simulink model "Demo1"  (Simulink 7.7)
settings: Solver=ode45  StartTime=0.0  StopTime=10  RelTol=1e-3
PreLoadFcn:
  | EbNo = 16; Errors = 188; Bits = 1e8; M = 256; N = 64; Ts = 1/22050; InnerInterleaverBitTable;constellation;
undefined symbols (not defined in the file or in its folder): gray, Rec, rsgenpoly, SDTV, sz
libraries: vipmisc x22, dspsigops x9, commutil2 x8, viptransforms x6, viputilities x6, vipconversions x4, dspobslib x4, commblkintrlv2 x4, commblkcod2 x2, vipsnks x2, commcnvintrlv2 x2, commsink2 x2
(part 2 of 2)

== system Demo1/Audio Source/Encoder/Block Processing/Block iterator/sub-block process/Transform coder2 ==
  In1 : Inport
  2D DCT : viptransforms/2-D DCT  CompMethod=Table lookup  Dimension=0  TableOpt=Speed  BitRevOrder=off  SkipNorm=off  firstCoeffDataTypeStr=Inherit: Same word length as input  firstCoeffLastDataTypeStr=Inherit: Same word length as input  outputMin=[]  outputMax=[]  roundingMode=Floor  overflowMode=off
  AC zigzag : Selector  IndexOptions=Index vector (dialog)  Indices="([0  8     1     2     9    16    24    17    10     3     4    11    18    25  32    40    33    26    19    12     5     6    13    20    27    34    41  48    56    49    42    35    28    21    14     7    15    22    29    36  43    50    57    58    51    44    37    30    23    31    38    45    52  59    60    53    46    39    47    54    61    62    55    63]+1)"  OutputSizes=1
  Bit Pack : Stateflow chart  TreatAsAtomicUnit=on
  Gain : Gain  Gain=255/8
  Gain1 : Gain  Gain=255/8
  Matrix Concatenation : Concatenate  Mode=Multidimensional array
  Reshape : Reshape  OutputDimensionality=Column vector (2-D)  OutputDimensions=[8,8]
  Reshape1 : Reshape  OutputDimensionality=Column vector (2-D)  OutputDimensions=[8,8]
  select 0 : Selector  IndexMode=Zero-based  IndexOptions=Index vector (dialog)  Indices=(0)  OutputSizes=8,8
  select 1 : Selector  IndexMode=Zero-based  IndexOptions=Starting index (dialog)  Indices=(1)  OutputSizes=63
  Out1 : Outport
  wires:
  Gain1/1 -> Matrix Concatenation/2
  select 1/1 -> Gain1/1
  Gain/1 -> Matrix Concatenation/1
  Matrix Concatenation/1 -> AC zigzag/1
  select 0/1 -> Gain/1
  Reshape/1 -> select 1/1, select 0/1
  Reshape1/1 -> Out1/1
  2D DCT/1 -> Reshape/1
  In1/1 -> 2D DCT/1
  AC zigzag/1 -> Bit Pack/1(in)
  Bit Pack/1(out) -> Reshape1/1

== system Demo1/Audio Sink/Decoder/Block Processing/Block iterator/sub-block process/Motion compensation decoder/SelectMatch3 ==
  Image : Inport
  Indx : Inport  Port=2
  Selector3 : Selector  NumberOfDimensions=2  IndexMode=Zero-based  InputPortWidth=3  IndexOptions=Starting index (port),Starting index (port)  Indices=1,1  OutputSizes=16, 16
  Selector4 : Selector  InputPortWidth=2  IndexOptions=Index vector (dialog)  Indices=1  OutputSizes=1
  Selector5 : Selector  InputPortWidth=2  IndexOptions=Index vector (dialog)  Indices=2  OutputSizes=1
  Out : Outport
  wires:
  Selector3/1 -> Out/1
  Indx/1 -> Selector5/1, Selector4/1
  Image/1 -> Selector3/1
  Selector5/1 -> Selector3/3
  Selector4/1 -> Selector3/2

== system Demo1/Audio Sink/Decoder/Block Processing/Block iterator/sub-block process/Motion compensation decoder/SelectMatch4 ==
  Image : Inport
  Indx : Inport  Port=2
  Selector3 : Selector  NumberOfDimensions=2  IndexMode=Zero-based  InputPortWidth=3  IndexOptions=Starting index (port),Starting index (port)  Indices=1,1  OutputSizes=8, 8
  Selector4 : Selector  InputPortWidth=2  IndexOptions=Index vector (dialog)  Indices=1  OutputSizes=1
  Selector5 : Selector  InputPortWidth=2  IndexOptions=Index vector (dialog)  Indices=2  OutputSizes=1
  Out : Outport
  wires:
  Selector4/1 -> Selector3/2
  Selector5/1 -> Selector3/3
  Image/1 -> Selector3/1
  Indx/1 -> Selector4/1, Selector5/1
  Selector3/1 -> Out/1

== system Demo1/Audio Sink/Decoder/Block Processing/Block iterator/sub-block process/Motion compensation decoder/SelectMatch5 ==
  Image : Inport
  Indx : Inport  Port=2
  Selector3 : Selector  NumberOfDimensions=2  IndexMode=Zero-based  InputPortWidth=3  IndexOptions=Starting index (port),Starting index (port)  Indices=1,1  OutputSizes=8, 8
  Selector4 : Selector  InputPortWidth=2  IndexOptions=Index vector (dialog)  Indices=1  OutputSizes=1
  Selector5 : Selector  InputPortWidth=2  IndexOptions=Index vector (dialog)  Indices=2  OutputSizes=1
  Out : Outport
  wires:
  Selector3/1 -> Out/1
  Indx/1 -> Selector5/1, Selector4/1
  Image/1 -> Selector3/1
  Selector5/1 -> Selector3/3
  Selector4/1 -> Selector3/2

== system Demo1/Audio Source/Encoder/Block Processing/Block iterator/sub-block process/Motion compensation encoder/SelectMatch ==
  Image : Inport
  Indx : Inport  Port=2
  Selector3 : Selector  NumberOfDimensions=2  IndexMode=Zero-based  InputPortWidth=3  IndexOptions=Starting index (port),Starting index (port)  Indices=(1),(1)  OutputSizes=16,16
  Selector4 : Selector  InputPortWidth=2  IndexOptions=Index vector (dialog)  Indices=(1)  OutputSizes=1
  Selector5 : Selector  InputPortWidth=2  IndexOptions=Index vector (dialog)  Indices=(2)  OutputSizes=1
  Out : Outport
  wires:
  Selector4/1 -> Selector3/2
  Selector5/1 -> Selector3/3
  Image/1 -> Selector3/1
  Indx/1 -> Selector4/1, Selector5/1
  Selector3/1 -> Out/1

== system Demo1/Audio Source/Encoder/Block Processing/Block iterator/sub-block process/Motion compensation encoder/SelectMatch1 ==
  Image : Inport
  Indx : Inport  Port=2
  Selector3 : Selector  NumberOfDimensions=2  IndexMode=Zero-based  InputPortWidth=3  IndexOptions=Starting index (port),Starting index (port)  Indices=(1),(1)  OutputSizes=8,8
  Selector4 : Selector  InputPortWidth=2  IndexOptions=Index vector (dialog)  Indices=(1)  OutputSizes=1
  Selector5 : Selector  InputPortWidth=2  IndexOptions=Index vector (dialog)  Indices=(2)  OutputSizes=1
  Out : Outport
  wires:
  Selector3/1 -> Out/1
  Indx/1 -> Selector5/1, Selector4/1
  Image/1 -> Selector3/1
  Selector5/1 -> Selector3/3
  Selector4/1 -> Selector3/2

== system Demo1/Audio Source/Encoder/Block Processing/Block iterator/sub-block process/Motion compensation encoder/SelectMatch2 ==
  Image : Inport
  Indx : Inport  Port=2
  Selector3 : Selector  NumberOfDimensions=2  IndexMode=Zero-based  InputPortWidth=3  IndexOptions=Starting index (port),Starting index (port)  Indices=(1),(1)  OutputSizes=8,8
  Selector4 : Selector  InputPortWidth=2  IndexOptions=Index vector (dialog)  Indices=(1)  OutputSizes=1
  Selector5 : Selector  InputPortWidth=2  IndexOptions=Index vector (dialog)  Indices=(2)  OutputSizes=1
  Out : Outport
  wires:
  Selector4/1 -> Selector3/2
  Selector5/1 -> Selector3/3
  Image/1 -> Selector3/1
  Indx/1 -> Selector4/1, Selector5/1
  Selector3/1 -> Out/1

== matlab function Audio Source/Encoder/Block Processing/Block iterator/sub-block process/Transform coder/Bit Pack ==
  data: in input double; out output uint32 size=20
function out=bitpack(in) 

% Pack output bits into given length using run length coding. The first 
% coefficient (DC) is coded using 32 bits. The AC coefficients are run 
% length coded using 4 bits for run and 8 bits for value. The output is uint32.

persistent prev_out;
if isempty(prev_out)
    prev_out = uint32(zeros(20,1));
end
    out=uint32(prev_out);
    % Bit Pack Routine  
    bitpos=int32(0); 
    Temp= uint32(0); 
    run =  uint32(0); 
    outpos = 2; 
    pval=single(0); 
    cval=single(0);
  
    numcoefs = 64;
    
    out1 =  int32(fix(in(1)));
    
    if out1>=-1   
       out(1) = uint32(out1);
    else
       out(1) = uint32(intmax('uint32') - uint32(abs(out1)) +uint32(2));
    end

    % ac coefficients
    % 4 bit - run length followed by 8 bit coef value  
    pval(:) = fix(in(2)+0.5);
    if (pval > 127),  pval(:) = 127; end % saturate  
    if (pval < -128), pval(:) = -128; end

    run(:) = 0;
    for i=(3): numcoefs   
        cval(:) = floor(in(i)+0.5); 
        if (pval == cval && run < 14)  
            run(:)=run(:)+1;
        else  
            [flag, bitpos, out, Temp, outpos] = putbits(bitpos, out, Temp, outpos, run, 4);
            if (~flag) 
                prev_out=out;
                return; 
            end

            if (pval > 127),  pval(:) = 127;  end % saturate  
            if (pval < -128), pval(:) = -128; end
            pval(:) = pval+128; % make positive  

            [flag, bitpos, out, Temp, outpos] = putbits(bitpos, out, Temp, outpos, uint32(pval), 8);
            if (~flag) 
                prev_out=out;
                return; 
            end

            run(:) = 0;
        end
        pval(:) = cval;
    end

    % last coefficient  
    [flag, bitpos, out, Temp, outpos] = putbits(bitpos, out, Temp, outpos, run, 4);
    if (~flag) 
        prev_out=out;
        return; 
    end

    if (pval > 127),  pval(:) = 127;  end % saturate 
    if (pval < -128), pval(:) = -128; end
    pval(:) = pval+128; % make positive 

    [flag, bitpos, out, Temp, outpos] = putbits(bitpos, out, Temp, outpos, pval, 8);
    if (~flag) 
        prev_out=out;
        return; 
    end

    [bitpos, out, Temp, outpos] = flushbits(bitpos, out, Temp, outpos);%#ok
    prev_out=out;
end

%%========================================================================
function [flag, bitposO, outO, TempO, outposO] = putbits(bitpos, out, Temp, outpos, val, bits)
     
    valIn = uint32(val);
    bitsIn=int32(bits);
    bitposO = int32(bitpos);
    outO = uint32(out);
    TempO = uint32(Temp);
    outposO = outpos;
    
    if (bitposO + bitsIn > 32)  
        bitsleft = int32(32 - bitposO);
        bval=uint32(0);
        bval(:) = bitshift(valIn, -(bitsIn-bitsleft)); 
        TempO(:) = bitor(TempO,bval); 
        outO(outposO) = TempO;
        outposO = outposO+1;
        if (outposO > length(out))  
            flag = 0;
            return;
        end
        TempO = uint32(0);
        bitposO(:) = int32(0);
        bitsIn(:) = bitsIn-bitsleft; 
        valIn(:)=bitshift(valIn, 32-bitsIn);  
        valIn(:)=bitshift(valIn, -(32-bitsIn)); 
    end
    valIn(:)=bitshift(valIn, (32-(bitsIn+(bitposO))));  
    TempO = bitor(TempO, valIn); 
    bitposO(:) = bitposO + bitsIn;
    flag=1;
end

%%========================================================================
function [bitposO, outO, TempO, outposO, out] = flushbits(bitpos, out, Temp, outpos)
 
    [flag, bitposO, outO, TempO, outposO] = putbits(bitpos, out, Temp, outpos, 15, 4);
    if (~flag) 
        return; 
    end
    if (outposO > length(out)+1), return; end
    outO(outposO) = TempO;
end

== matlab function Audio Sink/Decoder/Block Processing/Block iterator/sub-block process/Transform decoder/Bit Unpack ==
  data: in input double; out output single size=64
function out=bitunpack(in)

% Unpack the bits packed by the bit pack block. If there are not enough 
% values in the packed stream the rest of the output is filled with zeros.

persistent prev_out;
if isempty(prev_out)
    prev_out = single(zeros(64,1));
end
    out = prev_out;
    cbits= int32(0); 
    inpos=2; 
    Temp = uint32(0); 
    run = uint32(0);
    val = uint32(0);
   
    numcoefs = 64;
    if bitget(in(1),32)%negative
        out(1)=-int32(intmax('uint32')- uint32(in(1))) - int32(1);
    else
        out(1)=int32(in(1));
    end
    
    % ac coefficients
    % 4 bit - run length followed by 8 bit coef value  
    i=2;
    while (i<=numcoefs)   
         
        [flag, cbits, inpos, Temp, run] = getbits(cbits, inpos, Temp, in, run, 4);
        if (~flag) 
            break; 
        end
        if (run == 15), break;   end % end of stream  
        
        [flag, cbits, inpos, Temp, val] = getbits(cbits, inpos, Temp, in, val, 8);
        if (~flag) 
            break; 
        end 
        
        for j= i: min(run+i, numcoefs)    
            out(j) = single(single(val)-128.0);  
        end
        i = i + double(run)+1;
    end

    % when we havent got all coefs in the stream 
    for i=i:numcoefs    
        out(i) = 0;
    end
    prev_out(:)=out;
end

%%=================================================
function [flag, cbitsO, inposO, TempO, valO] = getbits(cbits, inpos, Temp, in, val, bits)

    lval = uint32(0); 
    temp = uint32(0);
    cbitsO = int32(cbits);
    inposO = inpos;
    TempO = uint32(Temp);
    valO = uint32(val);
    inwidth = length(in);
    if (cbitsO < bits)  
        if (inposO > inwidth) 
            flag=0;
            return; 
        end

        lval(:) =  bitshift(TempO, -(32-cbitsO));  
        bits(:) = bits - cbitsO;
        TempO = in(inposO); inposO = inposO +1;  
        lval = bitshift(lval, bits);  
        cbitsO(:) = int32(32);
    end

    temp(:) = bitshift(TempO, -(32-bits));  
    TempO(:) = bitshift(TempO, bits);  
    valO(:) = bitor(lval, temp); 
    cbitsO(:) = cbitsO - bits;

    flag = 1;
end

== matlab function Audio Sink/Decoder/Block Processing/Block iterator/sub-block process/Transform decoder1/Bit Unpack ==
  data: in input double; out output single size=64
function out=bitunpack(in)

% Unpack the bits packed by the bit pack block. If there are not enough 
% values in the packed stream the rest of the output is filled with zeros.

persistent prev_out;
if isempty(prev_out)
    prev_out = single(zeros(64,1));
end
    out = prev_out;
    cbits= int32(0); 
    inpos=2; 
    Temp = uint32(0); 
    run = uint32(0);
    val = uint32(0);
   
    numcoefs = 64;
    if bitget(in(1),32)%negative
        out(1)=-int32(intmax('uint32')- uint32(in(1))) - int32(1);
    else
        out(1)=int32(in(1));
    end
    
    % ac coefficients
    % 4 bit - run length followed by 8 bit coef value  
    i=2;
    while (i<=numcoefs)   
         
        [flag, cbits, inpos, Temp, run] = getbits(cbits, inpos, Temp, in, run, 4);
        if (~flag) 
            break; 
        end
        if (run == 15), break;   end % end of stream  
        
        [flag, cbits, inpos, Temp, val] = getbits(cbits, inpos, Temp, in, val, 8);
        if (~flag) 
            break; 
        end 
        
        for j= i: min(run+i, numcoefs)    
            out(j) = single(single(val)-128.0);  
        end
        i = i + double(run)+1;
    end

    % when we havent got all coefs in the stream 
    for i=i:numcoefs    
        out(i) = 0;
    end
    prev_out(:)=out;
end

%%=================================================
function [flag, cbitsO, inposO, TempO, valO] = getbits(cbits, inpos, Temp, in, val, bits)

    lval = uint32(0); 
    temp = uint32(0);
    cbitsO = int32(cbits);
    inposO = inpos;
    TempO = uint32(Temp);
    valO = uint32(val);
    inwidth = length(in);
    if (cbitsO < bits)  
        if (inposO > inwidth) 
            flag=0;
            return; 
        end

        lval(:) =  bitshift(TempO, -(32-cbitsO));  
        bits(:) = bits - cbitsO;
        TempO = in(inposO); inposO = inposO +1;  
        lval = bitshift(lval, bits);  
        cbitsO(:) = int32(32);
    end

    temp(:) = bitshift(TempO, -(32-bits));  
    TempO(:) = bitshift(TempO, bits);  
    valO(:) = bitor(lval, temp); 
    cbitsO(:) = cbitsO - bits;

    flag = 1;
end

== matlab function Audio Sink/Decoder/Block Processing/Block iterator/sub-block process/Transform decoder2/Bit Unpack ==
  data: in input double; out output single size=64
function out=bitunpack(in)

% Unpack the bits packed by the bit pack block. If there are not enough 
% values in the packed stream the rest of the output is filled with zeros.

persistent prev_out;
if isempty(prev_out)
    prev_out = single(zeros(64,1));
end
    out = prev_out;
    cbits= int32(0); 
    inpos=2; 
    Temp = uint32(0); 
    run = uint32(0);
    val = uint32(0);
   
    numcoefs = 64;
    if bitget(in(1),32)%negative
        out(1)=-int32(intmax('uint32')- uint32(in(1))) - int32(1);
    else
        out(1)=int32(in(1));
    end
    
    % ac coefficients
    % 4 bit - run length followed by 8 bit coef value  
    i=2;
    while (i<=numcoefs)   
         
        [flag, cbits, inpos, Temp, run] = getbits(cbits, inpos, Temp, in, run, 4);
        if (~flag) 
            break; 
        end
        if (run == 15), break;   end % end of stream  
        
        [flag, cbits, inpos, Temp, val] = getbits(cbits, inpos, Temp, in, val, 8);
        if (~flag) 
            break; 
        end 
        
        for j= i: min(run+i, numcoefs)    
            out(j) = single(single(val)-128.0);  
        end
        i = i + double(run)+1;
    end

    % when we havent got all coefs in the stream 
    for i=i:numcoefs    
        out(i) = 0;
    end
    prev_out(:)=out;
end

%%=================================================
function [flag, cbitsO, inposO, TempO, valO] = getbits(cbits, inpos, Temp, in, val, bits)

    lval = uint32(0); 
    temp = uint32(0);
    cbitsO = int32(cbits);
    inposO = inpos;
    TempO = uint32(Temp);
    valO = uint32(val);
    inwidth = length(in);
    if (cbitsO < bits)  
        if (inposO > inwidth) 
            flag=0;
            return; 
        end

        lval(:) =  bitshift(TempO, -(32-cbitsO));  
        bits(:) = bits - cbitsO;
        TempO = in(inposO); inposO = inposO +1;  
        lval = bitshift(lval, bits);  
        cbitsO(:) = int32(32);
    end

    temp(:) = bitshift(TempO, -(32-bits));  
    TempO(:) = bitshift(TempO, bits);  
    valO(:) = bitor(lval, temp); 
    cbitsO(:) = cbitsO - bits;

    flag = 1;
end

== matlab function Audio Source/Encoder/Block Processing/Block iterator/sub-block process/Transform coder1/Bit Pack ==
  data: in input double; out output uint32 size=20
function out=bitpack(in) 

% Pack output bits into given length using run length coding. The first 
% coefficient (DC) is coded using 32 bits. The AC coefficients are run 
% length coded using 4 bits for run and 8 bits for value. The output is uint32.

persistent prev_out;
if isempty(prev_out)
    prev_out = uint32(zeros(20,1));
end
    out=uint32(prev_out);
    % Bit Pack Routine  
    bitpos=int32(0); 
    Temp= uint32(0); 
    run =  uint32(0); 
    outpos = 2; 
    pval=single(0); 
    cval=single(0);
  
    numcoefs = 64;
    
    out1 =  int32(fix(in(1)));
    
    if out1>=-1   
       out(1) = uint32(out1);
    else
       out(1) = uint32(intmax('uint32') - uint32(abs(out1)) +uint32(2));
    end

    % ac coefficients
    % 4 bit - run length followed by 8 bit coef value  
    pval(:) = fix(in(2)+0.5);
    if (pval > 127),  pval(:) = 127; end % saturate  
    if (pval < -128), pval(:) = -128; end

    run(:) = 0;
    for i=(3): numcoefs   
        cval(:) = floor(in(i)+0.5); 
        if (pval == cval && run < 14)  
            run(:)=run(:)+1;
        else  
            [flag, bitpos, out, Temp, outpos] = putbits(bitpos, out, Temp, outpos, run, 4);
            if (~flag) 
                prev_out=out;
                return; 
            end

            if (pval > 127),  pval(:) = 127;  end % saturate  
            if (pval < -128), pval(:) = -128; end
            pval(:) = pval+128; % make positive  

            [flag, bitpos, out, Temp, outpos] = putbits(bitpos, out, Temp, outpos, uint32(pval), 8);
            if (~flag) 
                prev_out=out;
                return; 
            end

            run(:) = 0;
        end
        pval(:) = cval;
    end

    % last coefficient  
    [flag, bitpos, out, Temp, outpos] = putbits(bitpos, out, Temp, outpos, run, 4);
    if (~flag) 
        prev_out=out;
        return; 
    end

    if (pval > 127),  pval(:) = 127;  end % saturate 
    if (pval < -128), pval(:) = -128; end
    pval(:) = pval+128; % make positive 

    [flag, bitpos, out, Temp, outpos] = putbits(bitpos, out, Temp, outpos, pval, 8);
    if (~flag) 
        prev_out=out;
        return; 
    end

    [bitpos, out, Temp, outpos] = flushbits(bitpos, out, Temp, outpos);%#ok
    prev_out=out;
end

%%========================================================================
function [flag, bitposO, outO, TempO, outposO] = putbits(bitpos, out, Temp, outpos, val, bits)
     
    valIn = uint32(val);
    bitsIn=int32(bits);
    bitposO = int32(bitpos);
    outO = uint32(out);
    TempO = uint32(Temp);
    outposO = outpos;
    
    if (bitposO + bitsIn > 32)  
        bitsleft = int32(32 - bitposO);
        bval=uint32(0);
        bval(:) = bitshift(valIn, -(bitsIn-bitsleft)); 
        TempO(:) = bitor(TempO,bval); 
        outO(outposO) = TempO;
        outposO = outposO+1;
        if (outposO > length(out))  
            flag = 0;
            return;
        end
        TempO = uint32(0);
        bitposO(:) = int32(0);
        bitsIn(:) = bitsIn-bitsleft; 
        valIn(:)=bitshift(valIn, 32-bitsIn);  
        valIn(:)=bitshift(valIn, -(32-bitsIn)); 
    end
    valIn(:)=bitshift(valIn, (32-(bitsIn+(bitposO))));  
    TempO = bitor(TempO, valIn); 
    bitposO(:) = bitposO + bitsIn;
    flag=1;
end

%%========================================================================
function [bitposO, outO, TempO, outposO, out] = flushbits(bitpos, out, Temp, outpos)
 
    [flag, bitposO, outO, TempO, outposO] = putbits(bitpos, out, Temp, outpos, 15, 4);
    if (~flag) 
        return; 
    end
    if (outposO > length(out)+1), return; end
    outO(outposO) = TempO;
end

== matlab function Audio Source/Encoder/Block Processing/Block iterator/sub-block process/Transform coder2/Bit Pack ==
  data: in input double; out output uint32 size=20
function out=bitpack(in) 

% Pack output bits into given length using run length coding. The first 
% coefficient (DC) is coded using 32 bits. The AC coefficients are run 
% length coded using 4 bits for run and 8 bits for value. The output is uint32.

persistent prev_out;
if isempty(prev_out)
    prev_out = uint32(zeros(20,1));
end
    out=uint32(prev_out);
    % Bit Pack Routine  
    bitpos=int32(0); 
    Temp= uint32(0); 
    run =  uint32(0); 
    outpos = 2; 
    pval=single(0); 
    cval=single(0);
  
    numcoefs = 64;
    
    out1 =  int32(fix(in(1)));
    
    if out1>=-1   
       out(1) = uint32(out1);
    else
       out(1) = uint32(intmax('uint32') - uint32(abs(out1)) +uint32(2));
    end

    % ac coefficients
    % 4 bit - run length followed by 8 bit coef value  
    pval(:) = fix(in(2)+0.5);
    if (pval > 127),  pval(:) = 127; end % saturate  
    if (pval < -128), pval(:) = -128; end

    run(:) = 0;
    for i=(3): numcoefs   
        cval(:) = floor(in(i)+0.5); 
        if (pval == cval && run < 14)  
            run(:)=run(:)+1;
        else  
            [flag, bitpos, out, Temp, outpos] = putbits(bitpos, out, Temp, outpos, run, 4);
            if (~flag) 
                prev_out=out;
                return; 
            end

            if (pval > 127),  pval(:) = 127;  end % saturate  
            if (pval < -128), pval(:) = -128; end
            pval(:) = pval+128; % make positive  

            [flag, bitpos, out, Temp, outpos] = putbits(bitpos, out, Temp, outpos, uint32(pval), 8);
            if (~flag) 
                prev_out=out;
                return; 
            end

            run(:) = 0;
        end
        pval(:) = cval;
    end

    % last coefficient  
    [flag, bitpos, out, Temp, outpos] = putbits(bitpos, out, Temp, outpos, run, 4);
    if (~flag) 
        prev_out=out;
        return; 
    end

    if (pval > 127),  pval(:) = 127;  end % saturate 
    if (pval < -128), pval(:) = -128; end
    pval(:) = pval+128; % make positive 

    [flag, bitpos, out, Temp, outpos] = putbits(bitpos, out, Temp, outpos, pval, 8);
    if (~flag) 
        prev_out=out;
        return; 
    end

    [bitpos, out, Temp, outpos] = flushbits(bitpos, out, Temp, outpos);%#ok
    prev_out=out;
end

%%========================================================================
function [flag, bitposO, outO, TempO, outposO] = putbits(bitpos, out, Temp, outpos, val, bits)
     
    valIn = uint32(val);
    bitsIn=int32(bits);
    bitposO = int32(bitpos);
    outO = uint32(out);
    TempO = uint32(Temp);
    outposO = outpos;
    
    if (bitposO + bitsIn > 32)  
        bitsleft = int32(32 - bitposO);
        bval=uint32(0);
        bval(:) = bitshift(valIn, -(bitsIn-bitsleft)); 
        TempO(:) = bitor(TempO,bval); 
        outO(outposO) = TempO;
        outposO = outposO+1;
        if (outposO > length(out))  
            flag = 0;
            return;
        end
        TempO = uint32(0);
        bitposO(:) = int32(0);
        bitsIn(:) = bitsIn-bitsleft; 
        valIn(:)=bitshift(valIn, 32-bitsIn);  
        valIn(:)=bitshift(valIn, -(32-bitsIn)); 
    end
    valIn(:)=bitshift(valIn, (32-(bitsIn+(bitposO))));  
    TempO = bitor(TempO, valIn); 
    bitposO(:) = bitposO + bitsIn;
    flag=1;
end

%%========================================================================
function [bitposO, outO, TempO, outposO, out] = flushbits(bitpos, out, Temp, outpos)
 
    [flag, bitposO, outO, TempO, outposO] = putbits(bitpos, out, Temp, outpos, 15, 4);
    if (~flag) 
        return; 
    end
    if (outposO > length(out)+1), return; end
    outO(outposO) = TempO;
end
